simulink model "expert_control"  (R2023a)
settings: Solver=VariableStepAuto  StartTime=0.0  StopTime=1  RelTol=1e-3
model workspace (MAT data in the model file):
  F_m = 25
  Kb = 1.3
  Ks = 1
  theta_1 = 0.1
  theta_2 = 0.3
  theta_m = 0.5
libraries: spsSampleandHoldLib x1
settings Model: Creator=hch  LastModifiedBy=hch

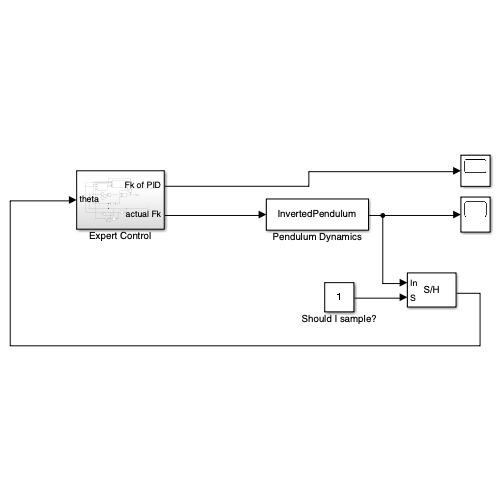
[thumbnail: Simulink's stored preview of the top-level diagram]
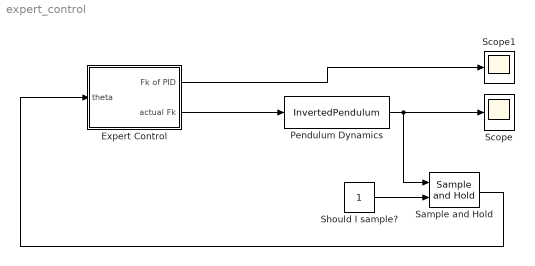
== system expert_control ==
  Expert Control : Subsystem
  Pendulum Dynamics : M-S-Function  FunctionName=InvertedPendulum  Parameters=pi/4,0,0,0
  Sample and Hold : spsSampleandHoldLib/Sample and Hold  ic=0  Ts=0.0001
      settings: LibrarySourceBlock=|
      | sps_lib/Control/Sample and
      | Hold
  Scope : Scope
  Scope1 : Scope
  Should I sample? : Constant
  wires:
  Pendulum Dynamics/1 -> Scope/1, Sample and Hold/1
  Should I sample?/1 -> Sample and Hold/2
  Sample and Hold/1 -> Expert Control/1(theta)
  Expert Control/1(Fk of PID) -> Scope1/1
  Expert Control/2(actual Fk) -> Pendulum Dynamics/1

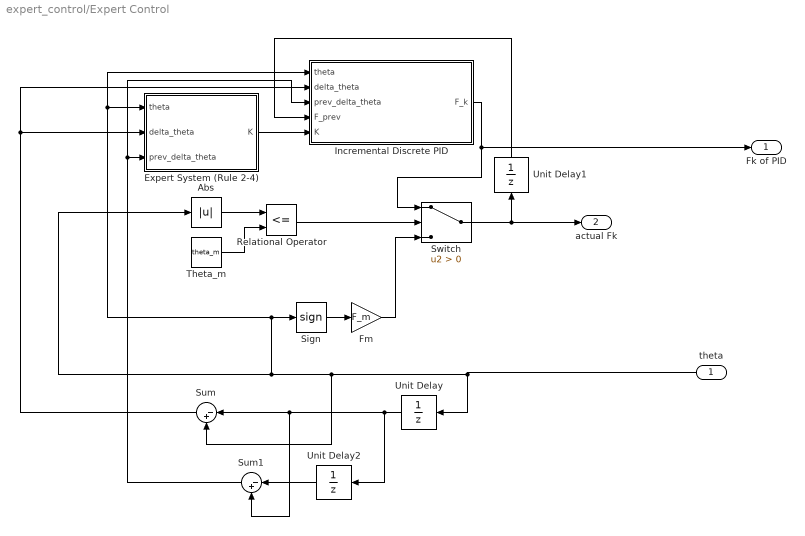
== system expert_control/Expert Control ==
  theta : Inport
  Abs : Abs  SaturateOnIntegerOverflow=off
  "Expert System (Rule 2-4) " : MATLAB Function  TreatAsAtomicUnit=on
  Fm : Gain  Gain=F_m
  Incremental Discrete PID : MATLAB Function  TreatAsAtomicUnit=on
  Relational Operator : RelationalOperator  Operator=<=  OutDataTypeStr=boolean  RndMeth=Simplest  InputSameDT=off
  Sign : Signum
  Sum : Sum  Inputs=|-+
  Sum1 : Sum  Inputs=|-+
  Switch : Switch  Criteria=u2 > Threshold  SaturateOnIntegerOverflow=off  InputSameDT=off
  Theta_m : Constant  Value=theta_m
  Unit Delay : UnitDelay  SampleTime=-1  HasFrameUpgradeWarning=on
  Unit Delay1 : UnitDelay  SampleTime=-1  HasFrameUpgradeWarning=on
  Unit Delay2 : UnitDelay  SampleTime=-1  HasFrameUpgradeWarning=on
  Fk of PID : Outport
  actual Fk : Outport  Port=2
  wires:
  Unit Delay2/1 -> Sum1/1
  Sign/1 -> Fm/1
  theta/1 -> Unit Delay/1, Sum/2, Abs/1, Incremental Discrete PID/1(theta), "Expert System (Rule 2-4) "/1(theta), Sign/1
  Sum1/1 -> "Expert System (Rule 2-4) "/3(prev_delta_theta), Incremental Discrete PID/3(prev_delta_theta)
  Abs/1 -> Relational Operator/1
  Theta_m/1 -> Relational Operator/2
  Unit Delay/1 -> Unit Delay2/1, Sum1/2, Sum/1
  Unit Delay1/1 -> Incremental Discrete PID/4(F_prev)
  Relational Operator/1 -> Switch/2
  Incremental Discrete PID/1(F_k) -> Fk of PID/1, Switch/1
  Sum/1 -> "Expert System (Rule 2-4) "/2(delta_theta), Incremental Discrete PID/2(delta_theta)
  "Expert System (Rule 2-4) "/1(K) -> Incremental Discrete PID/5(K)
  Fm/1 -> Switch/3
  Switch/1 -> actual Fk/1, Unit Delay1/1

== matlab function expert_control/Expert Control/Expert System (Rule 2-4)  ==
  data: theta input; K output; delta_theta input; prev_delta_theta input; theta_1 parameter; theta_2 parameter; theta_m parameter; Kb parameter; Ks parameter
function K = expert_system_rule(theta, delta_theta, prev_delta_theta, theta_1, theta_2, theta_m, Kb, Ks)

    % Initialize output
    K = 1; % Default K value

    % Rule (2): theta_2 <= |theta(k)| < theta_m
    if abs(theta) >= theta_2 && abs(theta) < theta_m
        if theta * delta_theta > 0
            K = Kb;
        elseif theta * delta_theta < 0
            if delta_theta * prev_delta_theta > 0
                K = 1;
            elseif delta_theta * prev_delta_theta < 0
                K = Kb;
            end
        end
        return;
    end

    % Rule (3): theta_1 <= |theta(k)| < theta_2
    if abs(theta) >= theta_1 && abs(theta) < theta_2
        if theta * delta_theta > 0
            K = 1;
        elseif theta * delta_theta < 0
            if delta_theta * prev_delta_theta > 0
                K = Ks;
            elseif delta_theta * prev_delta_theta < 0
                K = 1;
            end
        end
        return;
    end

    % Rule (4): |theta(k)| < theta_1
    if abs(theta) < theta_1
        K = 1;
    end
end

== matlab function expert_control/Expert Control/Incremental Discrete PID ==
  data: theta input; delta_theta input; F_k output; prev_delta_theta input; F_prev input; K input; F_m parameter
function F_k = incremental_pid(theta, delta_theta, prev_delta_theta, F_prev, K, F_m)
    % Declare parameters as constants
    % If these need to be dynamic, declare as inputs or global variables
    T = 0.0001;       % Sampling time
    Kp = 200;         % Proportional gain
    Ti = 0.001;       % Integral time
    Td = 10;          % Derivative time

    % Incremental PID formula
    F_k = F_prev + K * ( ...
        Kp * delta_theta + ...
        (T / Ti) * theta + ...
        (Td / T) * (delta_theta - prev_delta_theta) ...
    );

    % Saturate output to ensure |F_k| <= Fm
    if abs(F_k) > F_m
        F_k = sign(F_k) * F_m;
    end
end
